simulink model "diff_equiations"  (R2020b)
settings: Solver=VariableStepAuto  StartTime=0.0  StopTime=10.0  RelTol=1e-3
values from neighbouring files (symbols this model uses):
  c = 2    [diff_equiations_code.m]    (also in spring_eq_code.m)
  k = 2    [diff_equiations_code.m]    (also in spring_eq_code.m = 100)
  m = 5    [diff_equiations_code.m]    (also in electric_vehicle_edit.m = 1500; spring_eq_code.m = 2)
settings Model: Creator=amnessa  LastModifiedBy=amnessa

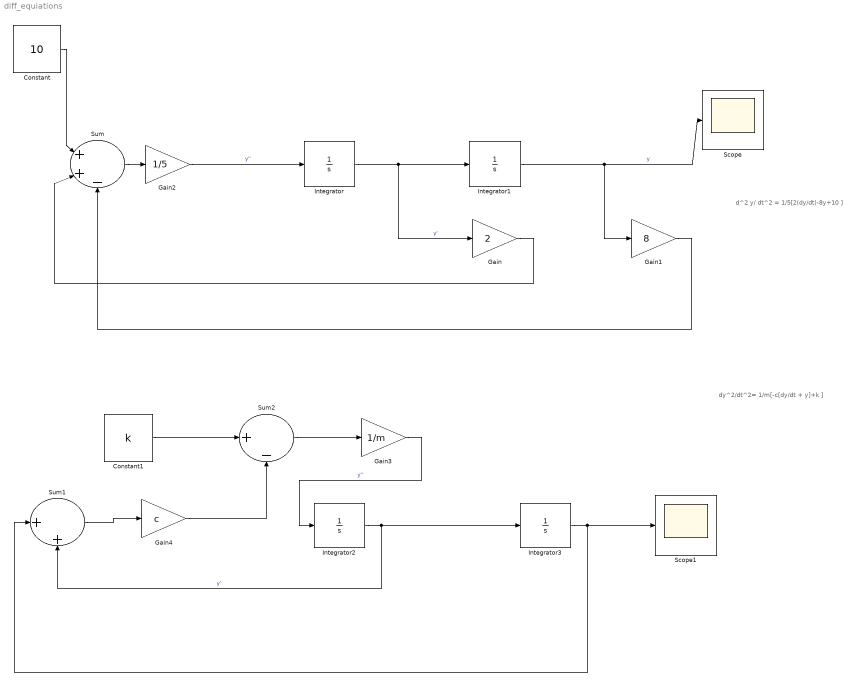
== system diff_equiations ==
  note: d^2 y/ dt^2 = 1/5[2(dy/dt)-8y+10 ]
  note: dy^2/dt^2= 1/m[-c[dy/dt + y]+k ]
  Constant : Constant  Value=10
  Constant1 : Constant  Value=k
  Gain : Gain  Gain=2
  Gain1 : Gain  Gain=8
  Gain2 : Gain  Gain=1/5
  Gain3 : Gain  Gain=1/m
  Gain4 : Gain  Gain=c
  Integrator{,1..3} (4 alike) : Integrator
  Scope : Scope
  Scope1 : Scope
  Sum : Sum  Inputs=|++-
  Sum1 : Sum  Inputs=|++
  Sum2 : Sum  Inputs=|+-
  wires:
  Sum/1 -> Gain2/1
  Gain2/1 -> Integrator/1  "y''"
  Integrator/1 -> Gain/1, Integrator1/1  "y'"
  Integrator1/1 -> Scope/1, Gain1/1  "y"
  Gain/1 -> Sum/2
  Gain1/1 -> Sum/3
  Constant/1 -> Sum/1
  Integrator2/1 -> Integrator3/1, Sum1/2  "y'"
  Integrator3/1 -> Sum1/1, Scope1/1
  Sum1/1 -> Gain4/1
  Gain4/1 -> Sum2/2
  Constant1/1 -> Sum2/1
  Sum2/1 -> Gain3/1
  Gain3/1 -> Integrator2/1  "y''"
